simulink model "StateSpace20240624SLX"  (R2023b)
settings: Solver=VariableStepAuto  StartTime=0.0  StopTime=10.0  RelTol=1e-3
values from neighbouring files (symbols this model uses):
  A = double(A)    [BolaIman.m]    (also in StateSpace20240624.m = [0 1;0 0])
  B = double(B)    [BolaIman.m]    (also in StateSpace20240624.m = [0;1])
  K = zpk([-1],0,.2)    [ScriptSimpleDiscretizacion20240617.m]    (also in StateSpace20240624.m = acker(A,B,[-2 -2]))
settings Model: Creator=AlejandroGhersin  LastModifiedBy=AlejandroGhersin

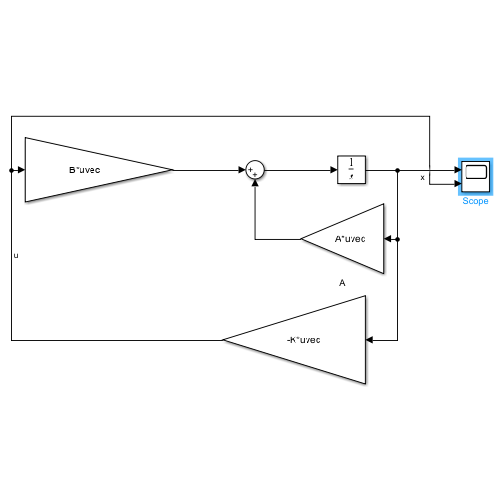
[thumbnail: Simulink's stored preview of the top-level diagram]
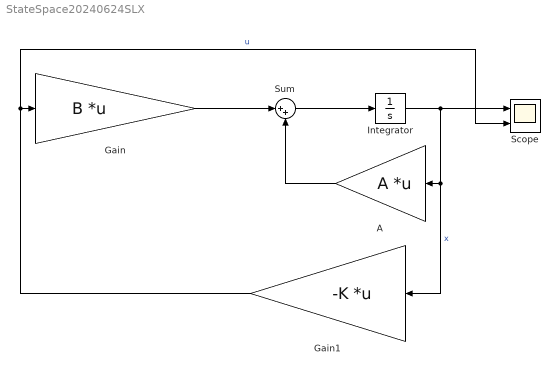
== system StateSpace20240624SLX ==
  A : Gain  Gain=A  Multiplication=Matrix(K*u) (u vector)
  Gain : Gain  Gain=B  Multiplication=Matrix(K*u) (u vector)
  Gain1 : Gain  Gain=-K  Multiplication=Matrix(K*u) (u vector)
  Integrator : Integrator  InitialCondition=[1;1]
  Scope : Scope  NumInputPorts=2
  Sum : Sum  Inputs=|++
  wires:
  Sum/1 -> Integrator/1
  Integrator/1 -> Gain1/1, A/1, Scope/1  "x"
  A/1 -> Sum/2
  Gain/1 -> Sum/1
  Gain1/1 -> Scope/2, Gain/1  "u"
